simulink model "TestAsset1"  (R2021a)
settings: Solver=VariableStepAuto  StartTime=0.0  StopTime=10  RelTol=1e-3
libraries: qss_tb_library x2, simulink x2
settings Model: Creator=egp
settings SolverCC: AlgebraicLoopSolver=TrustRegion
settings DataIOCC: ReturnWorkspaceOutputs=off
settings DebuggingCC: ArithmeticOperatorsInVariantConditions=warning
settings SFSimCC: SimUseLocalCustomCode=off  CustomCodeUndefinedFunction=UseInterfaceOnly
settings RTWCC: RTWUseLocalCustomCode=off  DLArmComputeVersion=20.02.1
settings ConfigComp: CovBoundaryAbsTol=1.0e-5

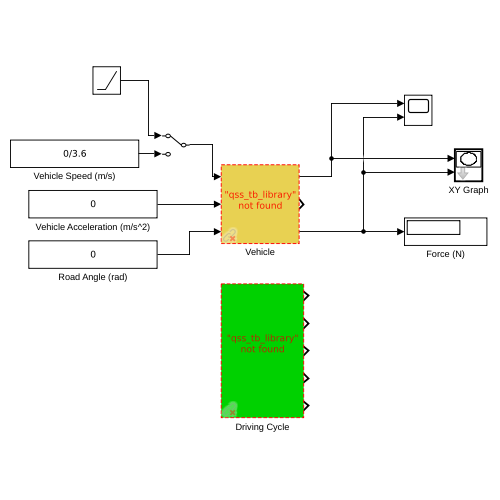
[thumbnail: Simulink's stored preview of the top-level diagram]
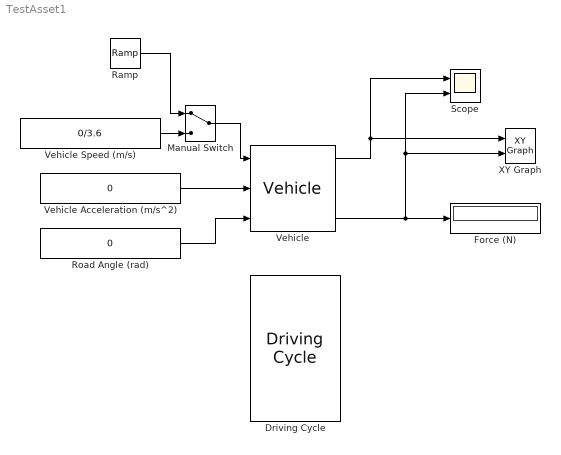
== system TestAsset1 ==
  Driving Cycle : qss_tb_library/Driving Cycle/Driving Cycle  Tag=cycle  cyclename1=NEDC  stepsize=1  autostop=on
  Force (N) : Display
  Manual Switch : ManualSwitch
  Ramp : simulink/Sources/Ramp  slope=60/3.6/10  start=0  InitialOutput=0
  Road Angle (rad) : Constant  Value=0
  Scope : Scope  NumInputPorts=2
  Vehicle : qss_tb_library/Vehicle/Vehicle  Tag=vehicle  m_f=1750  A_f=2.88  cw=0.5  mu=0.01  k_inertia=5
  Vehicle Acceleration (m/s^2) : Constant  Value=0
  Vehicle Speed (m/s) : Constant  Value=0/3.6
  XY Graph : simulink/Sinks/XY Graph  xmin=-1  xmax=1  ymin=-1  ymax=1  st=-1
  wires:
  Road Angle (rad)/1 -> Vehicle/3
  Vehicle Acceleration (m/s^2)/1 -> Vehicle/2
  Vehicle/3 -> XY Graph/2, Scope/2, Force (N)/1
  Vehicle Speed (m/s)/1 -> Manual Switch/2
  Ramp/1 -> Manual Switch/1
  Manual Switch/1 -> Vehicle/1
  Vehicle/1 -> XY Graph/1, Scope/1
